simulink model "Main_Topology_Final_Version"  (R2018a)
settings: Solver=FixedStepAuto  StartTime=0.0  StopTime=12  FixedStep=1e-5  RelTol=1e-3
libraries: powerlib x19, powerlib_meascontrol x2
settings Model: Creator=ASUS  LastModifiedBy=ASUS

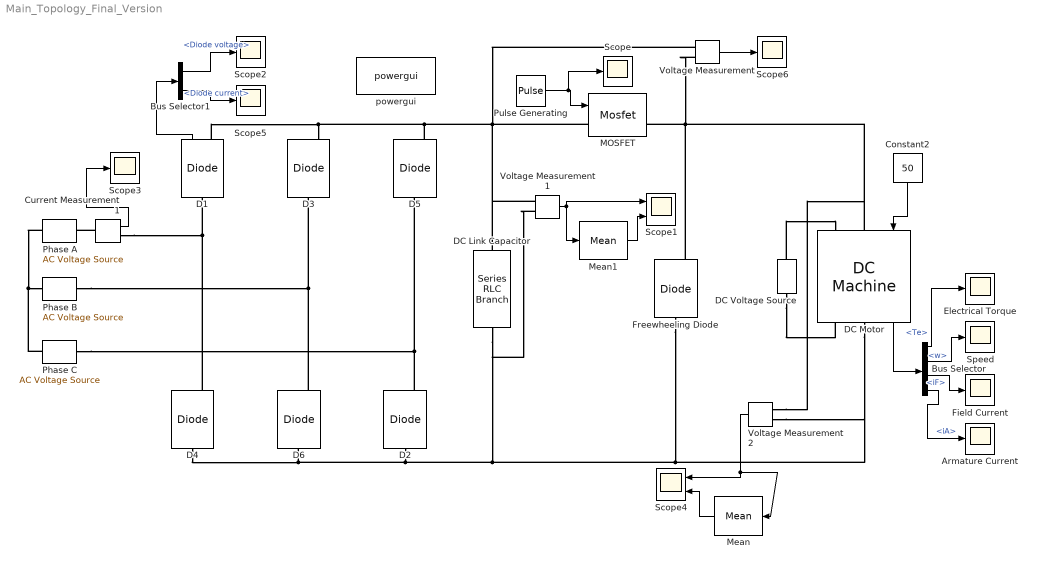
== system Main_Topology_Final_Version ==
  Armature Current : Scope
  Bus Selector : BusSelector  OutputSignals=Te,w,iF,iA
  Bus Selector1 : BusSelector  OutputSignals=Diode voltage,Diode current
  Constant2 : Constant  Value=50
  Current Measurement1 : powerlib/Measurements/Current Measurement  PhasorSimulation=off  OutputType=Complex  PSBequivalent=0
  D{1..6} (6 alike) : powerlib/Power Electronics/Diode  Ron=0.001  Lon=0  Vf=0.8  IC=0  UseSnubber=0  Rs=500  Cs=250e-9  Measurements=on
  DC Link Capacitor : powerlib/Elements/Series RLC Branch  LConnTagsString=__new0  RConnTagsString=__new0  BranchType=C  Resistance=1  Inductance=1e-3  SetiL0=off  InitialCurrent=0  Capacitance=1e-4  Setx0=on  InitialVoltage=200  Measurements=None
  DC Motor : powerlib/Machines/DC Machine  PresetModel=No  MechanicalLoad=Torque TL  FieldType=Wound  ShowDetailedParameters=on  MeasurementBus=on  RLa="[ 0.8  0.0125]"  RLf="[ 210  23]"  Laf=5  MachineConstant=Torque constant (N.m/A)  Ke=1.8  Kt=1.8  J=20  Bm=0  Tf=0  w0=0  Ifinit=1  TsPowergui=0  TsBlock=1e-4
  DC Voltage Source : powerlib/Electrical Sources/DC Voltage Source  Amplitude=140  Measurements=None
  Electrical Torque : Scope
  Field Current : Scope
  Freewheeling Diode : powerlib/Power Electronics/Diode  Ron=0.001  Lon=0  Vf=0.8  IC=0  UseSnubber=0  Rs=500  Cs=250e-9  Measurements=on
  MOSFET : powerlib/Power Electronics/Mosfet  Ron=0.1  Lon=0  Rd=0.01  Vfd=0  IC=0  Rs=1e5  Cs=inf  Measurements=on
  Mean : powerlib_meascontrol/Measurements/Mean  Freq=25  Vinit=0  Ts=0
  Mean1 : powerlib_meascontrol/Measurements/Mean  Freq=50  Vinit=0  Ts=0
  Phase A : powerlib/Electrical Sources/AC Voltage Source  Amplitude=90*sqrt(2)  Phase=0  Frequency=50  SampleTime=0  Measurements=None  BusType=swing  Pref=10e3  Qref=0  Qmin=-inf  Qmax=+inf
  Phase B : powerlib/Electrical Sources/AC Voltage Source  Amplitude=90*sqrt(2)  Phase=120  Frequency=50  SampleTime=0  Measurements=None  BusType=swing  Pref=10e3  Qref=0  Qmin=-inf  Qmax=+inf
  Phase C : powerlib/Electrical Sources/AC Voltage Source  Amplitude=90*sqrt(2)  Phase=240  Frequency=50  SampleTime=0  Measurements=None  BusType=swing  Pref=10e3  Qref=0  Qmin=-inf  Qmax=+inf
  Pulse Generating : DiscretePulseGenerator  PulseType=Time based  Period=4e-2  PulseWidth=10
  Scope{,2..3,5..6} (5 alike) : Scope
  Scope1 : Scope  NumInputPorts=2
  Scope4 : Scope  NumInputPorts=2
  Speed : Scope
  Voltage Measurement : powerlib/Measurements/Voltage Measurement  PhasorSimulation=off  OutputType=Complex  PSBequivalent=0
  Voltage Measurement1 : powerlib/Measurements/Voltage Measurement  PhasorSimulation=off  OutputType=Complex  PSBequivalent=0
  Voltage Measurement2 : powerlib/Measurements/Voltage Measurement  PhasorSimulation=off  OutputType=Complex  PSBequivalent=0
  powergui : powerlib/powergui  Priority=1  SimulationMode=Discrete  SampleTime=50e-6  frequency=60  Iterations=50  frequencyindice=0  Pbase=100e6  ErrMax=1e-4  UnitsV=kV  UnitsW=MW  buscounter=0  FunctionMessages=off  echomessages=off  EnableUseOfTLC=off  CurrentSourceSwitches=off  DisableSnubberDevices=off  DisableRonSwitches=off  DisableVfSwitches=off  DisplayEquations=off  SolverType=Tustin/Backward Euler (TBE)  Interpol=off  ExternalGateDelay=off  methode=off  Ts=100  x0status=blocks  SPID=off  SwTol=0  HookPort=off  RestoreLinks=warning  ResistiveCurrentMeasurement=off  Frange=[0:2:500]  Ylog=off  Xlog=on  ShowGrid=off  save=off  variable=ZData  structure=0  ZoomFFT=off  StartTime=0.0  cycles=1  DisplayStyle=1  fundamental=60  FreqAxis=off  MaxFrequency=1000  frequencyindicesteady=1  RmsSteady=1  display=off
  wires:
  Pulse Generating/1 -> Scope/1, MOSFET/1
  Mean1/1 -> Scope1/2
  Voltage Measurement1/1 -> Mean1/1, Scope1/1
  Constant2/1 -> DC Motor/1
  DC Motor/1 -> Bus Selector/1
  Bus Selector/1 -> Electrical Torque/1  "<Te>"
  Bus Selector/2 -> Speed/1  "<w>"
  Bus Selector/3 -> Field Current/1  "<iF>"
  Bus Selector/4 -> Armature Current/1  "<iA>"
  Voltage Measurement2/1 -> Mean/1, Scope4/1
  Current Measurement1/1 -> Scope3/1
  D1/1 -> Bus Selector1/1
  Bus Selector1/1 -> Scope2/1  "<Diode voltage>"
  Bus Selector1/2 -> Scope5/1  "<Diode current>"
  Voltage Measurement/1 -> Scope6/1
  Mean/1 -> Scope4/2
  connections:
  D4/RConn1 -- Current Measurement1/RConn1 -- D1/LConn1
  D6/RConn1 -- Phase B/RConn1 -- D3/LConn1
  D2/RConn1 -- Phase C/RConn1 -- D5/LConn1
  Phase A/LConn1 -- Phase C/LConn1 -- Phase B/LConn1
  D1/RConn1 -- Voltage Measurement1/LConn1 -- DC Link Capacitor/LConn1 -- Voltage Measurement/LConn1 -- MOSFET/LConn1 -- D5/RConn1 -- D3/RConn1
  Freewheeling Diode/LConn1 -- Voltage Measurement2/LConn2 -- DC Motor/RConn1 -- Voltage Measurement1/LConn2 -- DC Link Capacitor/RConn1 -- D2/LConn1 -- D4/LConn1 -- D6/LConn1
  Freewheeling Diode/RConn1 -- Voltage Measurement2/LConn1 -- DC Motor/LConn1 -- Voltage Measurement/LConn2 -- MOSFET/RConn1
  Current Measurement1/LConn1 -- Phase A/RConn1
  DC Voltage Source/RConn1 -- DC Motor/LConn2
  DC Voltage Source/LConn1 -- DC Motor/RConn2
